simulink model "NXT_Harness"  (R2018b)
settings: Solver=FixedStepDiscrete  StartTime=0.0  StopTime=20.0  FixedStep=0.2  RelTol=1e-3
undefined symbols (not defined in the file or in its folder): sigbuilder_block
settings Model: Creator=tony  LastModifiedBy=tony
settings OptimizationCC: BlockReduction=off
settings DebuggingCC: ConsistencyChecking=error  SignalInfNanChecking=error  SignalRangeChecking=error  AlgebraicLoopMsg=error  SigSpecEnsureSampleTimeMsg=error  IntegerOverflowMsg=error  ParameterUnderflowMsg=error  ParameterPrecisionLossMsg=error  ParameterTunabilityLossMsg=error  SFcnCompatibilityMsg=error  BusObjectLabelMismatch=error  RootOutportRequireBusObject=error  AllowSymbolicDim=off  ModelReferenceVersionMismatchMessage=error  ModelReferenceIOMismatchMessage=error  UnknownTsInhSupMsg=error  StrictBusMsg=ErrorOnBusTreatedAsVector  BusNameAdapt=ErrorWithoutRepair  NonBusSignalsTreatedAsBus=error  SFInvalidInputDataAccessInChartInitDiag=error  SFTransitionOutsideNaturalParentDiag=error  SFUnreachableExecutionPathDiag=error  SFExecutionAtInitializationDiag=error  SFMachineParentedDataDiag=error  IntegerSaturationMsg=error  AllowAutomaticUnitConversions=off
settings SFSimCC: SimUseLocalCustomCode=off  SimParseCustomCode=off

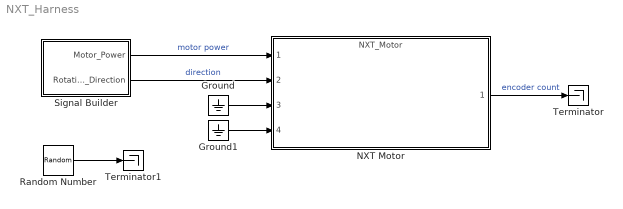
== system NXT_Harness ==
  Ground : Ground
  Ground1 : Ground
  NXT Motor : ModelReference  ModelNameDialog=NXT_Motor  SimulationMode=Normal  ModelReferenceVersion=1.13
  Random Number : RandomNumber  Variance=5  Seed=randi(1000)
  Signal Builder : Subsystem  Tag=STV Subsys  LoadFcn=sigbuilder_block('load');  StartFcn=sigbuilder_block('start');  StopFcn=sigbuilder_block('stop');  ClipboardFcn=sigbuilder_block('clipboard');  mask(Sigbuilder block){tuvar=[0:10]}
      mask help: Simulink:masks:SigbuilderBlock_MD
      mask init:
      | if ~strcmp(get_param(bdroot(gcbh),'SimulationStatus'),'stopped') tuvar = sigbuilder_block('maskInit'); end
      settings: CopyFcn=sigbuilder_block('copy');  DeleteFcn=sigbuilder_block('delete');  ModelCloseFcn=sigbuilder_block('modelClose');  PreSaveFcn=sigbuilder_block('preSave');  PauseFcn=sigbuilder_block('pause');  ContinueFcn=sigbuilder_block('continue');  NameChangeFcn=sigbuilder_block('namechange');  OpenFcn=sigbuilder_block('open',[364.547 27.2842 585.853 698.021 ]);  CloseFcn=sigbuilder_block('close');
      mask Display: plot(0, 0, 100, 100,[2, 2, 32, 32, 2], [68, 8, 8, 68, 68],[32, 2], [38, 38], [32, 19, 2],[53, 60, 44], [32, 17, 17, 2],[16, 16, 31, 31]);txt = getActiveGroup(gcbh);text(2, 100, txt,'verticalAlignment', 'top');
  Terminator : Terminator
  Terminator1 : Terminator
  wires:
  NXT Motor/1 -> Terminator/1  "encoder count"
  Signal Builder/1(Motor_Power) -> NXT Motor/1  "motor power"
  Signal Builder/2(Rotation_Direction) -> NXT Motor/2  "direction"
  Ground/1 -> NXT Motor/3
  Ground1/1 -> NXT Motor/4
  Random Number/1 -> Terminator1/1

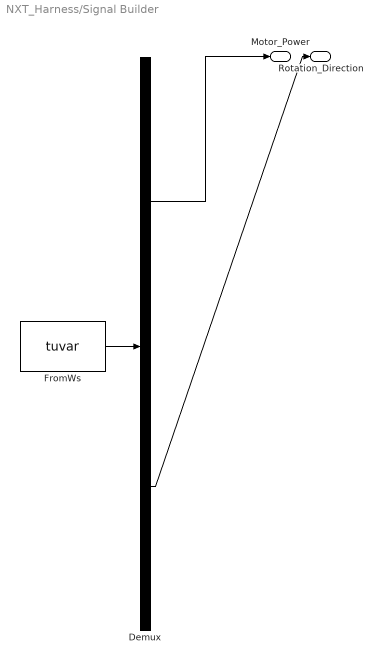
== system NXT_Harness/Signal Builder ==
  Demux : Demux  Tag=STV Demux  Outputs=2
  FromWs : FromWorkspace  Tag=STV FromWs  VariableName=tuvar  SampleTime=0.2
      SigBuilderData=|
      | common.afterFinalStr = 'Extrapolate'
      | common.sampleTime = '0.2'
      | dataSet(1).timeRange = [0 10]
      | dataSet(1).name = 'Two Step'
      | dataSet(2).timeRange = [0 10]
      | dataSet(2).name = 'Doublet'
      | sbobj.Groups(1).Name = 'Two Step'
      | sbobj.Groups(1).Signals(1).Name = 'Motor_Power'
      | sbobj.Groups(1).Signals(1).XData = [0 1 1 3 3 5 5 7 7 10]
      | sbobj.Groups(1).Signals(1).YData = [0 0 1 1 0 0 1 1 0 0]
      | sbobj.Groups(1).Signals(2).Name = 'Rotation_Direction'
      | sbobj.Groups(1).Signals(2).XData = [0 10]
      | sbobj.Groups(1).Signals(2).YData = [1 1]
      | sbobj.Groups(2).Name = 'Doublet'
      | sbobj.Groups(2).Signals(1).Name = 'Motor_Power'
      | sbobj.Groups(2).Signals(1).XData = [0 1 1 3 5 7 7 10]
      | sbobj.Groups(2).Signals(1).YData = [0 0 1 1 1 1 0 0]
      | sbobj.Groups(2).Signals(2).Name = 'Rotation_Direction'
      | sbobj.Groups(2).Signals(2).XData = [0 4 4 10]
      | sbobj.Groups(2).Signals(2).YData = [1 1 -1 -1]
  Motor_Power : Outport  Tag=STV Outport
  Rotation_Direction : Outport  Tag=STV Outport  Port=2
  wires:
  Demux/1 -> Motor_Power/1
  FromWs/1 -> Demux/1
  Demux/2 -> Rotation_Direction/1
